simulink model "observador_multirate_3"  (R2012b)
settings: Solver=ode3  StartTime=0.0  StopTime=10  FixedStep=1e-4  MaxStep=1e-4  RelTol=1e-3
values from neighbouring files (symbols this model uses):
  A = [-0.2  0; 1  0]    [teste_AxBu_AxBuLy_cadaumcomsuataxaindividual.mat]    (also in testes2.mat)
  B = [10 0]    [teste_AxBu_AxBuLy_cadaumcomsuataxaindividual.mat]    (also in testes2.mat)
  C = [0 1]    [teste_AxBu_AxBuLy_cadaumcomsuataxaindividual.mat]    (also in testes2.mat)
libraries: simulink x2, Encoder x1
settings Model: Creator=Juliano  LastModifiedBy=Juliano
settings DataIOCC: LimitDataPoints=off

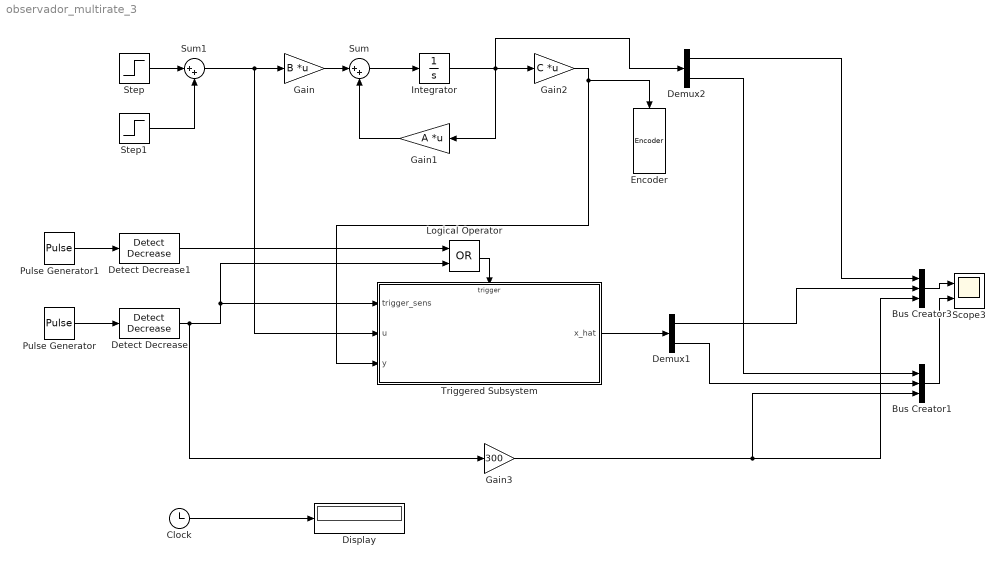
== system observador_multirate_3 ==
  Bus Creator1 : BusCreator  Inputs=3
  Bus Creator3 : BusCreator  Inputs=3
  Clock : Clock
  Demux1 : Demux  Outputs=2
  Demux2 : Demux  Outputs=2
  Detect Decrease : simulink/Logic and Bit Operations/Detect Decrease  vinit=0.0  InputProcessing=Inherited  OutDataTypeStr=boolean
  Detect Decrease1 : simulink/Logic and Bit Operations/Detect Decrease  vinit=0.0  InputProcessing=Inherited  OutDataTypeStr=boolean
  Display : Display
  Encoder : Encoder/Encoder  Nr=10
  Gain : Gain  Gain=B  Multiplication=Matrix(K*u)
  Gain1 : Gain  Gain=A  Multiplication=Matrix(K*u)
  Gain2 : Gain  Gain=C  Multiplication=Matrix(K*u)
  Gain3 : Gain  Gain=300  OutDataTypeStr=double
  Integrator : Integrator
  Logical Operator : Logic  Operator=OR  AllPortsSameDT=off  OutDataTypeStr=boolean
  Pulse Generator : DiscretePulseGenerator  PulseType=Time based  Period=1  PulseWidth=50
  Pulse Generator1 : DiscretePulseGenerator  PulseType=Time based  Period=0.03  PulseWidth=50
  Scope3 : Scope  NumInputPorts=2
      settings: ShowLegends=on  TimeRange=10  YMin=-35000~-5  YMax=50000~5  SaveName=ScopeData2
  Step : Step  Time=0  After=20  SampleTime=0
  Step1 : Step  Time=5  After=-40  SampleTime=0
  Sum : Sum  Inputs=|++
  Sum1 : Sum  Inputs=|++
  Triggered Subsystem : Subsystem  TreatAsAtomicUnit=on
  wires:
  Gain/1 -> Sum/1
  Gain1/1 -> Sum/2
  Sum/1 -> Integrator/1
  Integrator/1 -> Demux2/1, Gain2/1, Gain1/1
  Step/1 -> Sum1/1
  Step1/1 -> Sum1/2
  Gain2/1 -> Encoder/1, Triggered Subsystem/3(y)
  Bus Creator3/1 -> Scope3/1
  Pulse Generator1/1 -> Detect Decrease1/1
  Demux2/1 -> Bus Creator3/1
  Sum1/1 -> Triggered Subsystem/2(u), Gain/1
  Logical Operator/1 -> Triggered Subsystem/Trigger
  Detect Decrease1/1 -> Logical Operator/1
  Detect Decrease/1 -> Gain3/1, Triggered Subsystem/1(trigger_sens), Logical Operator/2
  Triggered Subsystem/1(x_hat) -> Demux1/1
  Demux1/1 -> Bus Creator3/2
  Pulse Generator/1 -> Detect Decrease/1
  Gain3/1 -> Bus Creator1/3, Bus Creator3/3
  Clock/1 -> Display/1
  Demux2/2 -> Bus Creator1/1
  Demux1/2 -> Bus Creator1/2
  Bus Creator1/1 -> Scope3/2

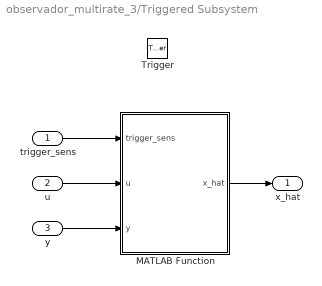
== system observador_multirate_3/Triggered Subsystem ==
  trigger_sens : Inport
  u : Inport  Port=2
  y : Inport  Port=3
  Trigger : TriggerPort
  MATLAB Function : MATLAB Function  TreatAsAtomicUnit=on
  x_hat : Outport
  wires:
  MATLAB Function/1(x_hat) -> x_hat/1
  y/1 -> MATLAB Function/3(y)
  u/1 -> MATLAB Function/2(u)
  trigger_sens/1 -> MATLAB Function/1(trigger_sens)

== matlab function observador_multirate_3/Triggered Subsystem/MATLAB Function ==
  data: trigger_sens input; u input; y input; x_hat output
function x_hat  = fcn(trigger_sens, u, y)
    %#codegen
    persistent Ts;
    persistent A;
    persistent B;
    persistent C;
    persistent D;
    persistent L;
    persistent measurement_flag;
    persistent x;

    if(isempty(Ts))
        % Define as matrizes.
        Ts = 0.03;
        A = [1-0.2*Ts 0 ; Ts 1];
        B = [10*Ts ; 0];
        C = [0 1];
        D = 0;
        L = [-0.18+0.2/Ts+0.04*Ts ; 0.9-0.2*Ts];

        measurement_flag = 0;
        x = [0;0];
    end


    if(trigger_sens == 1)
        measurement_flag = 1;
    else
        if(measurement_flag == 0)
            x = A*x+B*u;
        else
            x = A*x+B*u+L*(y-C*x);
            measurement_flag = 0;
        end
    end

    x_hat = x;

end
